simulink model "MatMul_Processor"  (R2023b)
settings: Solver=VariableStepAuto  StartTime=0.0  StopTime=10.0  RelTol=1e-3
settings Model: Creator=lenovo GAME  LastModifiedBy=lenovo GAME

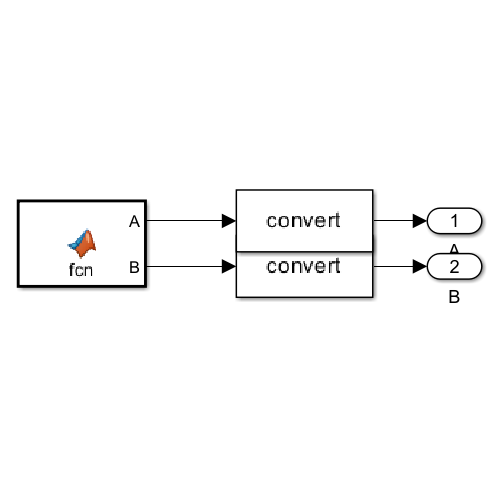
[thumbnail: Simulink's stored preview of the top-level diagram]
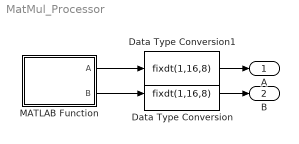
== system MatMul_Processor ==
  Data Type Conversion : DataTypeConversion  OutDataTypeStr=fixdt(1,16,8)  SaturateOnIntegerOverflow=off  RndMeth=Floor
  Data Type Conversion1 : DataTypeConversion  OutDataTypeStr=fixdt(1,16,8)  SaturateOnIntegerOverflow=off  RndMeth=Floor
  MATLAB Function : MATLAB Function  TreatAsAtomicUnit=on
  A : Outport
  B : Outport  Port=2
  wires:
  MATLAB Function/1(A) -> Data Type Conversion1/1
  MATLAB Function/2(B) -> Data Type Conversion/1
  Data Type Conversion1/1 -> A/1
  Data Type Conversion/1 -> B/1

== matlab function MatMul_Processor/MATLAB Function ==
  data: A output; B output
function [A, B] = fcn()
Amat = [1 2 3; 4 5 6; 7 8 9];
Bmat = [9 8 7; 6 5 4; 3 2 1];
A = Amat(:);   % 9x1
B = Bmat(:);   % 9x1
end
